simulink model "heli_q8_copy"  (R2016b)
settings: Solver=ode1  StartTime=0.0  StopTime=inf  FixedStep=0.002  RelTol=1e-3  EnableMultiTasking=on
PostLoadFcn:
  | qc_set_target_type(getConfigSet(bdroot, 'QUARC Default Target Configuration'));
values from neighbouring files (symbols this model uses):
  k1 = (l_p*k_f)/(j_p)    (= 0.611111111111)    [P2p1_init.m]    (also in P2p2_init.m; init_heli_all.m)
  k2 = ((k_f*l_h)/(j_e))    (= 0.0983420026008)    [P2p1_init.m]    (also in P2p2_init.m; init_heli_all.m)
  k_pd = (2*zeta * omega0)/k1    (= 7.7111819679)    [P2p1_init.m]    (also in P2p2_init.m; init_heli_all.m)
  k_pp = (omega0^2)/k1    (= 9.08452223282)    [P2p1_init.m]    (also in P2p2_init.m; init_heli_all.m)
  k_rp = -1.0    (= -1)    [P2p1_init.m]    (also in P2p2_init.m; init_heli_all.m)
settings Model: SimulationMode=external  ExtModeTrigDuration=5000  Creator=Rchan  LastModifiedBy=Kevin K. Kaldvansvik
settings SolverCC: PositivePriorityOrder=on
settings DataIOCC: LimitDataPoints=on  SaveFormat=Array  SignalLoggingSaveFormat=ModelDataLogs
settings OptimizationCC: ExpressionDepthLimit=2147483647  InitFltsAndDblsToZero=on  LifeSpan=inf
settings DebuggingCC: SaveWithParameterizedLinksMsg=none  UnderspecifiedInitializationDetection=Classic  MergeDetectMultiDrivingBlocksExec=none  SolverPrmCheckMsg=warning  MultiTaskDSMMsg=warning  MultiTaskCondExecSysMsg=none  FcnCallInpInsideContextMsg=warning  StateNameClashWarn=warning  SFUnexpectedBacktrackingDiag=warning  SFNoUnconditionalDefaultTransitionDiag=warning  SFExecutionAtInitializationDiag=none
settings HardwareCC: ProdBitPerPointer=32  ProdBitPerSizeT=32  ProdBitPerPtrDiffT=32  ProdLargestAtomicFloat=None  ProdIntDivRoundTo=Undefined  ProdEndianess=Unspecified  ProdWordSize=32  ProdHWDeviceType=32-bit Generic
settings ModelReferenceCC: PropagateSignalLabelsOutOfModel=off
settings RTWCC: SystemTargetFile=quarc_win64.tlc  TemplateMakefile=quarc_default_tmf  Description=QUARC Win64 Target
settings STFCustomTargetCC: TargetPreCompLibLocation=C:\PROGRA~3\QUARC\lib\2014a\win64\release  ConcurrentExecutionCompliant=on  GeneratePreprocessorConditionals=Disable all  CPPClassGenCompliant=on  SystemTargetFile=quarc_win64.tlc
settings GRTTargetCC: TargetPreCompLibLocation=C:\PROGRA~3\QUARC\lib\2014a\win64\release  TargetLangStandard=C89/C90 (ANSI)  ParMdlRefBuildCompliant=off  CompOptLevelCompliant=off  GeneratePreprocessorConditionals=Disable all  CombineOutputUpdateFcns=off  MatFileLogging=off  GRTInterface=on  UseToolchainInfoCompliant=off  ExtMode=on  ExtModeMexFile=quarc_comm
settings ConfigComp: CovMetricSettings=dw  CovHtmlReporting=on  CovSaveCumulativeToWorkspaceVar=on  CovSaveSingleToWorkspaceVar=on  CovExternalEMLEnable=off  CovSFcnEnable=off

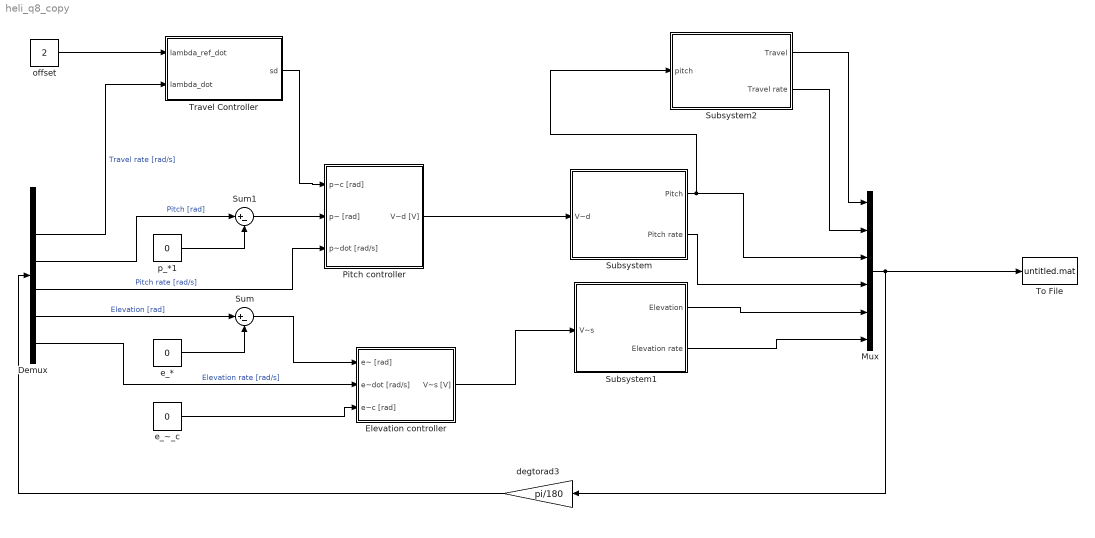
== system heli_q8_copy ==
  Demux : Demux  Outputs=6
  Elevation controller : Subsystem
  Mux : Mux  Inputs=6
  Pitch controller : Subsystem
  Subsystem : Subsystem
  Subsystem1 : Subsystem
  Subsystem2 : Subsystem
  Sum : Sum  Inputs=|+-
  Sum1 : Sum  Inputs=|+-
  To File : ToFile  MatrixName=kp_v1
  Travel Controller : Subsystem
  degtorad3 : Gain  Gain=pi/180
  e_* : Constant  Value=0
  e_~_c : Constant  Value=0
  offset : Constant  Value=2
  p_*1 : Constant  Value=0
  wires:
  e_~_c/1 -> Elevation controller/3(e~c [rad])
  e_*/1 -> Sum/2
  Demux/6 -> Elevation controller/2(e~dot [rad/s])  "Elevation rate [rad/s]"
  Sum/1 -> Elevation controller/1(e~ [rad])
  p_*1/1 -> Sum1/2
  Sum1/1 -> Pitch controller/2(p~ [rad])
  Demux/4 -> Pitch controller/3(p~dot [rad/s])  "Pitch rate [rad/s]"
  Mux/1 -> degtorad3/1, To File/1
  degtorad3/1 -> Demux/1
  Demux/5 -> Sum/1  "Elevation [rad]"
  Demux/3 -> Sum1/1  "Pitch [rad]"
  Demux/2 -> Travel Controller/2("lambda_dot ")  "Travel rate [rad/s]"
  Travel Controller/1("sd ") -> Pitch controller/1(p~c [rad])
  offset/1 -> Travel Controller/1("lambda_ref_dot ")
  Pitch controller/1(V~d [V]) -> Subsystem/1(V~d)
  Subsystem/1(Pitch) -> Subsystem2/1(pitch), Mux/3
  Subsystem/2(Pitch rate) -> Mux/4
  Elevation controller/1(V~s [V]) -> Subsystem1/1(V~s)
  Subsystem1/1(Elevation) -> Mux/5
  Subsystem1/2(Elevation rate) -> Mux/6
  Subsystem2/1(Travel) -> Mux/1
  Subsystem2/2(Travel rate) -> Mux/2

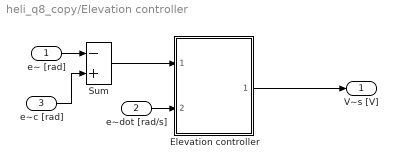
== system heli_q8_copy/Elevation controller ==
  e~ [rad] : Inport
  e~dot [rad/s] : Inport  Port=2
  e~c [rad] : Inport  Port=3
  Elevation controller : Subsystem
  Sum : Sum  Inputs=-+  SaturateOnIntegerOverflow=on  InputSameDT=on  OutDataTypeStr=Inherit: Same as first input
  V~s [V] : Outport  InitialOutput=0
  wires:
  Sum/1 -> Elevation controller/1(e~ [rad])
  Elevation controller/1(V~_s [V]) -> V~s [V]/1
  e~ [rad]/1 -> Sum/1
  e~dot [rad/s]/1 -> Elevation controller/2(e~_dot [rad/s])
  e~c [rad]/1 -> Sum/2

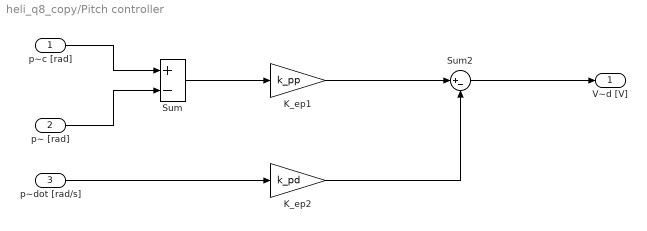
== system heli_q8_copy/Pitch controller ==
  p~c [rad] : Inport
  p~ [rad] : Inport  Port=2
  p~dot [rad/s] : Inport  Port=3
  K_ep1 : Gain  Gain=k_pp  SaturateOnIntegerOverflow=on  OutDataTypeStr=Inherit: Same as input  ParamDataTypeStr=Inherit: Same as input
  K_ep2 : Gain  Gain=k_pd  SaturateOnIntegerOverflow=on  OutDataTypeStr=Inherit: Same as input  ParamDataTypeStr=Inherit: Same as input
  Sum : Sum  Inputs=+-  SaturateOnIntegerOverflow=on  InputSameDT=on  OutDataTypeStr=Inherit: Same as first input
  Sum2 : Sum  Inputs=|+-
  V~d [V] : Outport  InitialOutput=0
  wires:
  p~c [rad]/1 -> Sum/1
  p~ [rad]/1 -> Sum/2
  Sum/1 -> K_ep1/1
  p~dot [rad/s]/1 -> K_ep2/1
  K_ep1/1 -> Sum2/1
  K_ep2/1 -> Sum2/2
  Sum2/1 -> V~d [V]/1

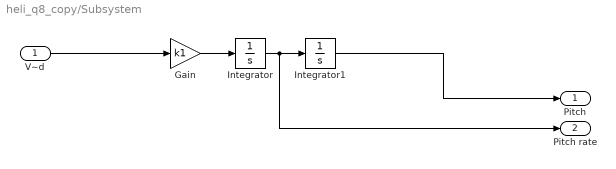
== system heli_q8_copy/Subsystem ==
  V~d : Inport
  Gain : Gain  Gain=k1
  Integrator : Integrator
  Integrator1 : Integrator
  Pitch : Outport
  Pitch rate : Outport  Port=2
  wires:
  Integrator/1 -> Pitch rate/1, Integrator1/1
  Integrator1/1 -> Pitch/1
  V~d/1 -> Gain/1
  Gain/1 -> Integrator/1

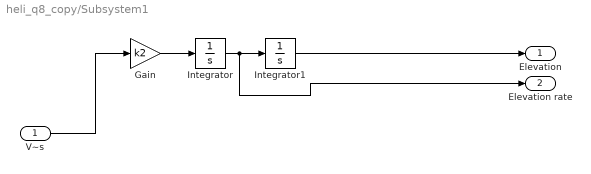
== system heli_q8_copy/Subsystem1 ==
  V~s : Inport
  Gain : Gain  Gain=k2
  Integrator : Integrator
  Integrator1 : Integrator
  Elevation : Outport
  Elevation rate : Outport  Port=2
  wires:
  Gain/1 -> Integrator/1
  Integrator/1 -> Elevation rate/1, Integrator1/1
  V~s/1 -> Gain/1
  Integrator1/1 -> Elevation/1

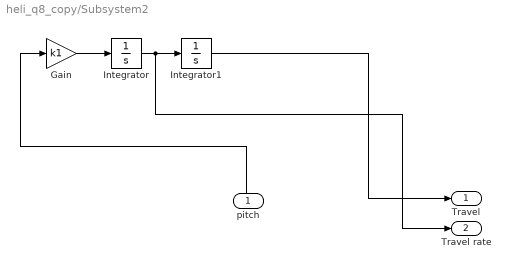
== system heli_q8_copy/Subsystem2 ==
  pitch : Inport
  Gain : Gain  Gain=k1
  Integrator : Integrator
  Integrator1 : Integrator
  Travel : Outport
  Travel rate : Outport  Port=2
  wires:
  Gain/1 -> Integrator/1
  Integrator1/1 -> Travel/1
  Integrator/1 -> Travel rate/1, Integrator1/1
  pitch/1 -> Gain/1

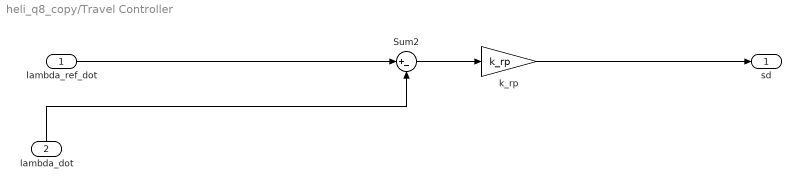
== system heli_q8_copy/Travel Controller ==
  "lambda_ref_dot " : Inport
  "lambda_dot " : Inport  Port=2
  Sum2 : Sum  Inputs=|+-
  k_rp : Gain  Gain=k_rp
  "sd " : Outport
  wires:
  k_rp/1 -> "sd "/1
  Sum2/1 -> k_rp/1
  "lambda_ref_dot "/1 -> Sum2/1
  "lambda_dot "/1 -> Sum2/2

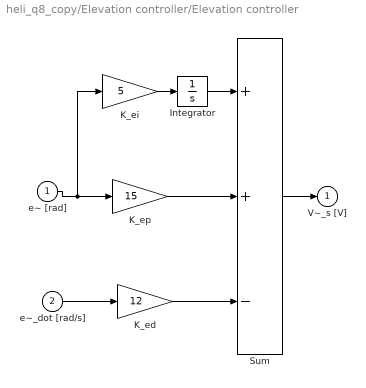
== system heli_q8_copy/Elevation controller/Elevation controller ==
  e~ [rad] : Inport
  e~_dot [rad/s] : Inport  Port=2
  Integrator : Integrator  LimitOutput=on
  K_ed : Gain  Gain=12  SaturateOnIntegerOverflow=on  OutDataTypeStr=Inherit: Same as input  ParamDataTypeStr=Inherit: Same as input
  K_ei : Gain  Gain=5  SaturateOnIntegerOverflow=on  OutDataTypeStr=Inherit: Same as input  ParamDataTypeStr=Inherit: Same as input
  K_ep : Gain  Gain=15  SaturateOnIntegerOverflow=on  OutDataTypeStr=Inherit: Same as input  ParamDataTypeStr=Inherit: Same as input
  Sum : Sum  Inputs=++-  SaturateOnIntegerOverflow=on  InputSameDT=on  OutDataTypeStr=Inherit: Same as first input
  V~_s [V] : Outport  InitialOutput=0
  wires:
  K_ei/1 -> Integrator/1
  Integrator/1 -> Sum/1
  Sum/1 -> V~_s [V]/1
  e~_dot [rad/s]/1 -> K_ed/1
  K_ed/1 -> Sum/3
  K_ep/1 -> Sum/2
  e~ [rad]/1 -> K_ep/1, K_ei/1
